simulink model "P2"  (R2015b)
settings: Solver=ode45  StartTime=0.0  StopTime=10.0  RelTol=1e-3
undefined symbols (not defined in the file): DiscIntNeverNeededParam
libraries: simulink x1, dspsrcs4 x1
settings Model: Creator=Augusto  LastModifiedBy=Jefferson
settings DataIOCC: SaveFormat=Array
settings DebuggingCC: SolverPrmCheckMsg=warning  AllowSymbolicDim=on
settings HardwareCC: ProdBitPerPointer=32  ProdLargestAtomicFloat=None  ProdIntDivRoundTo=Undefined  ProdEndianess=Unspecified  ProdWordSize=32  ProdHWDeviceType=32-bit Generic
settings GRTTargetCC: GeneratePreprocessorConditionals=Disable all
settings ConfigComp: CovModelRefEnable=Off  CovSFcnEnable=off

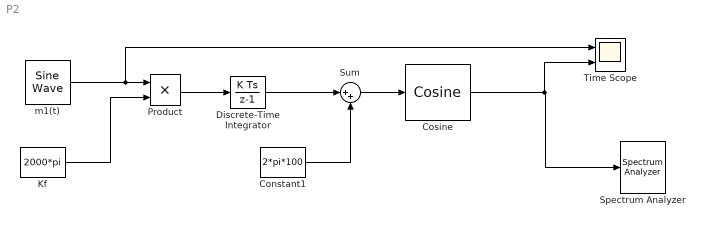
== system P2 ==
  Constant1 : Constant  Value=2*pi*100
  Cosine : simulink/Lookup Tables/Cosine  Formula=cos(2*pi*u)  NumDataPoints=(2^5)+1  OutputWordLength=16  InternalRulePriority=Speed
  Discrete-Time Integrator : DiscreteIntegrator  InitialConditionSetting=State (most efficient)  SampleTime=-1  ICPrevOutput=DiscIntNeverNeededParam  ICPrevScaledInput=DiscIntNeverNeededParam
  "Kf " : Constant  Value=2000*pi
  Product : Product
  Spectrum Analyzer : SpectrumAnalyzer
  Sum : Sum  Inputs=|++
  Time Scope : Scope  NumInputPorts=2
  "m1(t) " : dspsrcs4/Sine Wave  Amplitude=1  Frequency=20  Phase=0  SampleMode=Discrete  OutComplex=Real  CompMethod=Trigonometric fcn  TableSize=Speed  SampleTime=1/5000  SamplesPerFrame=1  ResetState=Restart at time zero  OutputFrames=on  dataType=double  wordLen=16  udDataType=sfix(16)  fracBitsMode=Best precision  numFracBits=15  OutDataTypeStr=double  LastOutDataTypeStr=double
  wires:
  "m1(t) "/1 -> Time Scope/1, Product/1
  "Kf "/1 -> Product/2
  Constant1/1 -> Sum/2
  Product/1 -> Discrete-Time Integrator/1
  Discrete-Time Integrator/1 -> Sum/1
  Sum/1 -> Cosine/1
  Cosine/1 -> Time Scope/2, Spectrum Analyzer/1
